simulink model "Gorev4"  (R2019b)
settings: Solver=ode45  StartTime=0.0  StopTime=500.0  RelTol=1e-3
settings Model: Creator=Bekircan Keceoglu  LastModifiedBy=Bekircan Keceoglu

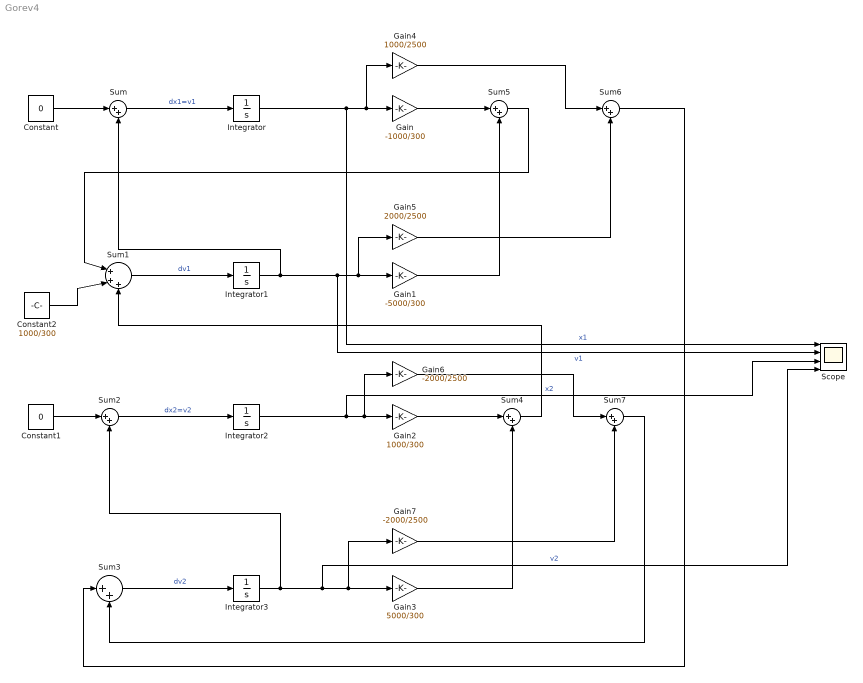
== system Gorev4 ==
  Constant : Constant  Value=0
  Constant1 : Constant  Value=0
  Constant2 : Constant  Value=1000/300
  Gain : Gain  Gain=-1000/300
  Gain1 : Gain  Gain=-5000/300
  Gain2 : Gain  Gain=1000/300
  Gain3 : Gain  Gain=5000/300
  Gain4 : Gain  Gain=1000/2500
  Gain5 : Gain  Gain=2000/2500
  Gain6 : Gain  Gain=-2000/2500
  Gain7 : Gain  Gain=-2000/2500
  Integrator : Integrator  InitialCondition=1
  Integrator1 : Integrator  InitialCondition=0.8
  Integrator2 : Integrator  InitialCondition=0.1
  Integrator3 : Integrator  InitialCondition=0.4
  Scope : Scope  NumInputPorts=4
  Sum{,2..7} (7 alike) : Sum  Inputs=|++
  Sum1 : Sum  Inputs=|+++
  wires:
  Sum/1 -> Integrator/1  "dx1=v1"
  Integrator/1 -> Scope/1, Gain4/1, Gain/1  "x1"
  Sum1/1 -> Integrator1/1  "dv1"
  Integrator1/1 -> Sum/2, Scope/2, Gain5/1, Gain1/1  "v1"
  Constant/1 -> Sum/1
  Sum2/1 -> Integrator2/1  "dx2=v2"
  Sum3/1 -> Integrator3/1  "dv2"
  Integrator3/1 -> Sum2/2, Scope/4, Gain7/1, Gain3/1  "v2"
  Constant1/1 -> Sum2/1
  Integrator2/1 -> Scope/3, Gain6/1, Gain2/1  "x2"
  Gain/1 -> Sum5/1
  Gain1/1 -> Sum5/2
  Sum5/1 -> Sum1/1
  Gain2/1 -> Sum4/1
  Gain3/1 -> Sum4/2
  Sum4/1 -> Sum1/3
  Gain4/1 -> Sum6/1
  Gain5/1 -> Sum6/2
  Gain6/1 -> Sum7/1
  Gain7/1 -> Sum7/2
  Sum6/1 -> Sum3/1
  Sum7/1 -> Sum3/2
  Constant2/1 -> Sum1/2
